simulink model "simulink_control"  (R2024a)
settings: Solver=ode5  StartTime=0.0  StopTime=inf  FixedStep=0.016  RelTol=1e-3
values from neighbouring files (symbols this model uses):
  accelerometer_sensor = wb_robot_get_device('accelerometer')    [simulink_control_app.m]
  alpha_pitch = 0.85    [simulink_control_app.m]
  gyro_sensor = wb_robot_get_device('gyro')    [simulink_control_app.m]
  inertial_unit = wb_robot_get_device('inertial_unit')    [simulink_control_app.m]
  left_rotational_motor = wb_robot_get_device('left_rotational_motor')    [simulink_control_app.m]
  right_rotational_motor = wb_robot_get_device('right_rotational_motor')    [simulink_control_app.m]
  TIME_STEP = 16    [simulink_control_app.m]
undefined symbols (not defined in the file or in its folder): A, B
libraries: simulink_extras x6, eeGeneralControl x3, simulink x3, robotmobilelib x1, embmathops x1
(part 2 of 2)

== matlab function simulink_control/Control Architecture/MATLAB Function ==
  data: params input; x input; u input; A output; B output; f output
function [A, B, f] = system_matrices(params, x, u)
    % Parameters
    k1 = params.k1;
    k2 = params.k2;
    m = params.m;
    n = params.n;
    
    A22 = -2 * k2 * (params.Mp * params.R * params.L^2 + params.Mp * params.R^2 * params.L + params.JPt * params.R) / m;
    A23 = -(params.Mp^2 * params.R^2 * params.L^2 * params.g) / m;
    A42 = -2 * k2 / (params.JPt + params.Mp * params.L);
    A43 = (params.Mp * params.g * params.L) / (params.JPt + params.Mp * params.L);
    A66 = -k2 * params.D^2 * params.R / n;

    % A Matrix
    A = [
        0, 1, 0, 0, 0, 0;
        0, A22, A23, 0, 0, 0;
        0, 0, 0, 1, 0, 0;
        0, A42, A43, 0, 0, 0;
        0, 0, 0, 0, 0, 1;
        0, 0, 0, 0, 0, A66;
    ];
    
    % B Matrix
    B21 = -k1 * params.D * params.R / (params.JPt + params.Mp * params.L);
    B62 = k1 * (params.Mp * params.R * params.L^2 + params.Mp * params.R^2 * params.L + params.JPt * params.R) / m;
    B = [
        0, 0;
        B21, 0;
        0, 0;
        0, 0;
        0, 0;
        0, B62;
    ];
    
    % Disturbance Vector f
    f = [0; params.f2; 0; params.f4; 0; params.f6];
end

== matlab function simulink_control/Control Architecture/MATLAB Function1 ==
  data: params output; x0 output; u1 input; u2 input; u output
function [params,x0,u] = fcn(u1,u2)
params.N = 100;
params.kt = 0.5;
params.ke = 0.3;
params.Ra = 2.0;
params.Mp = 0.5;
params.g = 9.81;
params.f2 = 0;
params.f4 = 0;
params.f6 = 0;

x0 = [0; 0; 0; 0; 0; 0]; 

u = [0.2; -0.1];

== matlab function simulink_control/Send Webots Simulation/MATLAB Function ==
  data: u input; y output
function y = fcn(u)

y = u;

== matlab function simulink_control/Control Architecture/Subsystem/MATLAB Function2 ==
  data: pid_output input; yaw_error input; motorSteering output; pitch_error input
function motorSteering = fcn_yaw_control(pid_output, yaw_error, pitch_error)
% Maksimum yönlendirme sınırları
max_steering = 25.0;

% Pitch hatasının etkisini hesapla (Eğer pitch hatası büyükse yönlendirme azaltılmalı)
pitch_sensitivity = max(0, 1 - abs(pitch_error) / 10); % 10 derece üzerinde yönlendirme azaltılır

% Yaw hatasının etkisini hesapla (Eğer yaw hatası büyükse yönlendirme artırılmalı)
yaw_sensitivity = max(0, 1 - abs(yaw_error) / 15); % 15 derece üzerinde yönlendirme azaltılır
if abs(pid_output) < 5
    motorSteering = 0; % Çok küçük hataları yok say
elseif abs(pid_output) < 15
    motorSteering = pid_output * 0.5 * pitch_sensitivity * yaw_sensitivity; % Orta dereceli düzeltme
else
    motorSteering = pid_output * pitch_sensitivity * yaw_sensitivity; % Büyük hatalarda tam kontrol
end

% Çıkışı sınırlama
motorSteering = max(-max_steering, min(max_steering, motorSteering));

end

== matlab function simulink_control/Control Architecture/Subsystem5/MATLAB Function3 ==
  settings: updateMethod=DISCRETE
  data: yaw_error input; pitch_error input; pid_output input; motorSteering output
function motorSteering = balanceControl(yaw_error, pitch_error, pid_output)
    % balanceControl: İki tekerlekli aracın denge ve yönlendirme kontrolünü sağlar.
    %
    % Girdiler:
    %   yaw_error: (desired_yaw - measured_yaw) olarak hesaplanan yaw hatası (derece)
    %   pitch_error: (desired_pitch - measured_pitch) olarak hesaplanan pitch hatası (derece)
    %   pid_output: Yaw kontrol PID çıkışı
    %
    % Çıktı:
    %   motorSteering: Direksiyon açısı (derece)

    % Pitch error sınırları
    min_pitch = -22;
    max_pitch = 22;
    
    % Eğer pitch error [-22, 22] arasında ise, PID çıkışını kullan, değilse 0 yap
    if pitch_error >= min_pitch && pitch_error <= max_pitch
        motorSteering = pid_output;
    else
        motorSteering = pid_output;
    end
end
